simulink model "prelab"  (R2021b)
settings: Solver=VariableStepAuto  StartTime=0.0  StopTime=10  RelTol=1e-3
values from neighbouring files (symbols this model uses):
  C = eye(4)    [lab5.m]    (also in lab5_2.m)
  D = [0;0;0;0]    [lab5.m]    (also in lab5_2.m)
  F1 = -1*place(A_a, B_a, [-1.5 -1.6 -1.7 -1.8])    [lab5.m]    (also in lab5_2.m)
  init_condit = [0;0;0;0]    [lab5.m]    (also in lab5_2.m)
undefined symbols (not defined in the file or in its folder): A_a, B_a
settings Model: Creator=varunsampat  LastModifiedBy=varunsampat

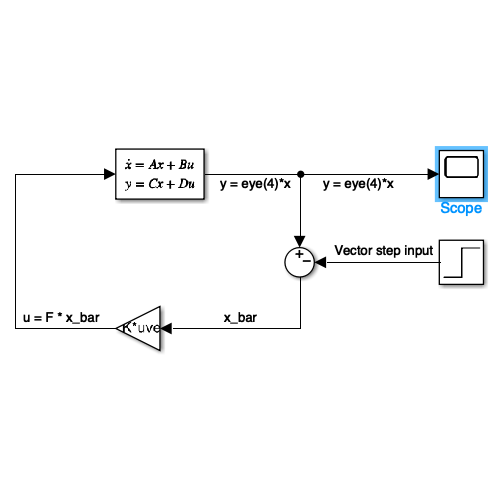
[thumbnail: Simulink's stored preview of the top-level diagram]
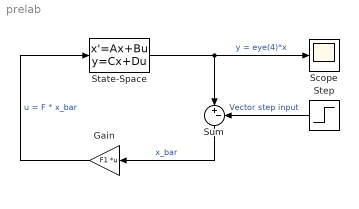
== system prelab ==
  Gain : Gain  Gain=F1  Multiplication=Matrix(K*u) (u vector)
  Scope : Scope
  State-Space : StateSpace  A=A_a  B=B_a  C=C  D=D  InitialCondition=init_condit
  Step : Step  Before=[0; 0; 0; 0]  After=[1; 0; 0; 0]  SampleTime=0
  Sum : Sum  Inputs=|+-
  wires:
  State-Space/1 -> Sum/1, Scope/1  "y = eye(4)*x"
  Sum/1 -> Gain/1  "x_bar"
  Gain/1 -> State-Space/1  "u = F * x_bar"
  Step/1 -> Sum/2  "Vector step input"
